simulink model "CryoDetMultiChan_CMB"  (R2016b)
settings: Solver=ode45  StartTime=0.0  StopTime=1000e-6  MaxStep=Tclk/4  RelTol=1e-3
values from neighbouring files (symbols this model uses):
  ds_axi = 16    [setupCryoFPGA_CMB.m]
  Fclk = Fadc    (= 307200000)    [setupCryoFPGA.m]    (also in setupCryoFPGA_CMB.m; setupCryoFPGAorig.m = 312500000)
  notch = tf( [1 a*wNotch/Q wNotch^2], [1 wNotch/Q wNotch^2])    [setupCryoFPGA.m]    (also in setupCryoFPGA_CMB.m; setupCryoFPGAorig.m)
  notch2 = tf( [1 a*wNotch/Q wNotch^2], [1 wNotch/Q wNotch^2])    [setupCryoFPGA.m]    (also in setupCryoFPGA_CMB.m; setupCryoFPGAorig.m)
  notch3 = tf( [1 a*wNotch/Q wNotch^2], [1 wNotch/Q wNotch^2])    [setupCryoFPGA.m]    (also in setupCryoFPGA_CMB.m; setupCryoFPGAorig.m)
  notch4 = tf( [1 a*wNotch/Q wNotch^2], [1 wNotch/Q wNotch^2])    [setupCryoFPGA.m]    (also in setupCryoFPGA_CMB.m; setupCryoFPGAorig.m)
  Tclk = 1/Fclk    (= 3.25520833333e-09)    [setupCryoFPGA.m]    (also in setupCryoFPGA_CMB.m; setupCryoFPGAorig.m = 3.2e-09)
  Ts = 1/Fadc    (= 3.25520833333e-09)    [setupCryoFPGA.m]    (also in setupCryoFPGA_CMB.m; setupCryoFPGAorig.m = 3.2e-09)
undefined symbols (not defined in the file or in its folder): AXI4, i, Lite, xlipgetpartsetting
libraries: xbsIndex_r4 x2077, CryoDetLib x32, hdlsllib x6, simulink x3
(part 11 of 15)

== system CryoDetMultiChan_CMB/DspCore/FTA_Ch0/SixteenLineUDC 0/oneLineUpDown2 ==
  note: `
  note: Delta-F
  note: When synchIn == Addr then reset CIC filters
  note: Turn off this channel if Frequency is 0 or Fnyquist
  note: first data comes out 31 ticks after release of reset
  note: should we tag data with channel number (from addr) and tvalid?
      | This could help synchronize (and debug) next stage decimator
  note: Latch phase advance for interleave at 1/614.4MHz
  note: Decimated_mxREF_QI
  note: Decimated_mxREF_Q
  note: Decimated_mxADC_I
  note: Decimated_mxADC_Q
  note: DAC 1
  note: DAC 0
  note: Downconverter
  note: Downmixed & Decmiated SIG & REF IQ to Output Mux for interleaving
  note: Phase CICs so outputs for different lines interleave; this is done so by timing the CIC reset operation between line channels
  note: 1/614.4MHz phase advance
  note: Digital LO for one resonator
  note: Upconverter
  note: Multiply Signal & Reference
      | by complex LO
      | Note: we don't need dPhi here b/c its not interleaved
  note: mixed_ADC_Q
  note: mixed_ADC_I
  note: mixed_REF_Q
  note: mixed_REF_I
  note: Address
  note: mixed_dec_ADC_IQ
  note: mixed_dec_REF_IQ
  note: LO + Phi Q
  note: LO + Phi I
  note: Complex multiply adds the phase advance to the output frequency per sample:
      |
      | e^jwt x e^jphi = e^j(wt+phi)
  note: Multipliers are for
      | Amplitude Scaling
  note: LO & LO+phi to DAC sum block
  ADC_IQ_in : Inport
  addrIn : Inport  Port=2
  synchIn : Inport  Port=3
  REF_IQ_in1 : Inport  Port=4
  Bus Creator : BusCreator  Inputs=4
  Bus Selector : BusSelector  OutputSignals=channel,dPhiQ,dPhiI
  CIC Compiler 4.0 {,1..3} (4 alike) : xbsIndex_r4/CIC Compiler 4.0   filter_type=Decimation  number_of_stages=3  differential_delay=1  number_of_channels=1  sample_rate_changes=Fixed  fixed_or_initial_rate=16  minimum_rate=16  maximum_rate=16  ratespecification=Sample_Period  sampleperiod=1  hardwareoversamplingrate=1  quantization=Truncation  output_data_width=20  use_xtreme_dsp_slice=off  use_streaming_interface=on  has_aclken=off  has_aresetn=on  has_dout_tready=off  trim_axipin_name=on  gui_behaviour=Sysgen_GUI  input_data_width=18  ip_name=CIC Compiler  ip_version=4.0  dsptool_ready=true  wrapper_available=true  port_translation_map={ 'aclken' => 'en', 'aresetn' => 'rst' }  ipcore_xco_need_fpga_part=true  ipcore_verbose=false  block_type=cic_compiler_v4_0
  Complex Multiplier 6.0 1 : xbsIndex_r4/Complex Multiplier 6.0   hasatlast=off  hasatuser=off  atuserwidth=1  hasbtlast=off  hasbtuser=off  btuserwidth=1  multtype=Use_Mults  optimizegoal=Resources  flowcontrol=NonBlocking  outputwidth=18  roundmode=Truncate  hasctrltlast=off  hasctrltuser=off  ctrltuserwidth=1  outtlastbehv=Null  latencyconfig=Manual  minimumlatency=6  aclken=off  aresetn=off  trim_axipin_name=on  simulation_type=hybrid_sim  simulation_model=sysgen:cmpy_v6_0  data_path_portlist={ 's_axis_a_tdata_real', 's_axis_a_tdata_imag', 's_axis_b_tdata_real', 's_axis_b_tdata_imag', 's_axis_ctrl_tdata_rounding_bit', 'm_axis_dout_tdata_real', 'm_axis_dout_tdata_imag' }  aportwidth=63  bportwidth=63  ip_name=Complex Multiplier  ip_version=6.0  dsptool_ready=true  ipcore_usecache=true  ipcore_useipmodelcache=true  ipcore_verbose=false  ipcore_latency_parameter='minimumlatency'  wrapper_available=true  port_translation_map={ 'aclken' => 'en', 'aresetn' => 'rst'}  block_type=cmpy_v6_0
  Complex Multiplier 6.0 2 : xbsIndex_r4/Complex Multiplier 6.0   hasatlast=off  hasatuser=off  atuserwidth=1  hasbtlast=off  hasbtuser=off  btuserwidth=1  multtype=Use_Mults  optimizegoal=Resources  flowcontrol=NonBlocking  outputwidth=18  roundmode=Truncate  hasctrltlast=off  hasctrltuser=off  ctrltuserwidth=1  outtlastbehv=Null  latencyconfig=Manual  minimumlatency=6  aclken=off  aresetn=off  trim_axipin_name=on  simulation_type=hybrid_sim  simulation_model=sysgen:cmpy_v6_0  data_path_portlist={ 's_axis_a_tdata_real', 's_axis_a_tdata_imag', 's_axis_b_tdata_real', 's_axis_b_tdata_imag', 's_axis_ctrl_tdata_rounding_bit', 'm_axis_dout_tdata_real', 'm_axis_dout_tdata_imag' }  aportwidth=63  bportwidth=63  ip_name=Complex Multiplier  ip_version=6.0  dsptool_ready=true  ipcore_usecache=true  ipcore_useipmodelcache=true  ipcore_verbose=false  ipcore_latency_parameter='minimumlatency'  wrapper_available=true  port_translation_map={ 'aclken' => 'en', 'aresetn' => 'rst'}  block_type=cmpy_v6_0
  Complex Multiplier 6.0 4 : xbsIndex_r4/Complex Multiplier 6.0   hasatlast=off  hasatuser=off  atuserwidth=1  hasbtlast=off  hasbtuser=off  btuserwidth=1  multtype=Use_Mults  optimizegoal=Resources  flowcontrol=NonBlocking  outputwidth=19  roundmode=Truncate  hasctrltlast=off  hasctrltuser=off  ctrltuserwidth=1  outtlastbehv=Null  latencyconfig=Manual  minimumlatency=6  aclken=off  aresetn=off  trim_axipin_name=on  simulation_type=hybrid_sim  simulation_model=sysgen:cmpy_v6_0  data_path_portlist={ 's_axis_a_tdata_real', 's_axis_a_tdata_imag', 's_axis_b_tdata_real', 's_axis_b_tdata_imag', 's_axis_ctrl_tdata_rounding_bit', 'm_axis_dout_tdata_real', 'm_axis_dout_tdata_imag' }  aportwidth=63  bportwidth=63  ip_name=Complex Multiplier  ip_version=6.0  dsptool_ready=true  ipcore_usecache=true  ipcore_useipmodelcache=true  ipcore_verbose=false  ipcore_latency_parameter='minimumlatency'  wrapper_available=true  port_translation_map={ 'aclken' => 'en', 'aresetn' => 'rst'}  block_type=cmpy_v6_0
  Constant : xbsIndex_r4/Constant  const=1  gui_display_data_type=Boolean  arith_type=Boolean  n_bits=16  bin_pt=14  preci_type=Single  exp_width=8  frac_width=24  explicit_period=on  period=Tclk  equ=P=C  opselect=C  inp2=PCIN>>17  opr=+  inp1=P  carry=CIN  dbl_ovrd=off  block_type=constant
  Constant1 : xbsIndex_r4/Constant  const=0  gui_display_data_type=Fixed-point  arith_type=Unsigned  n_bits=16  bin_pt=16  preci_type=Single  exp_width=8  frac_width=24  explicit_period=off  period=1  equ=P=C  opselect=C  inp2=PCIN>>17  opr=+  inp1=P  carry=CIN  dbl_ovrd=off  block_type=constant
  Constant2 : xbsIndex_r4/Constant  const=0  gui_display_data_type=Fixed-point  arith_type=Unsigned  n_bits=16  bin_pt=16  preci_type=Single  exp_width=8  frac_width=24  explicit_period=off  period=1  equ=P=C  opselect=C  inp2=PCIN>>17  opr=+  inp1=P  carry=CIN  dbl_ovrd=off  block_type=constant
  Constant3 : xbsIndex_r4/Constant  const=1  gui_display_data_type=Boolean  arith_type=Boolean  n_bits=16  bin_pt=14  preci_type=Single  exp_width=8  frac_width=24  explicit_period=on  period=Tclk  equ=P=C  opselect=C  inp2=PCIN>>17  opr=+  inp1=P  carry=CIN  dbl_ovrd=off  block_type=constant
  Convert1 : xbsIndex_r4/Convert  gui_display_data_type=Fixed-point  arith_type="Signed  (2's comp)"  n_bits=16  bin_pt=14  float_type=Single  exp_bits=8  fraction_bits=24  quantization=Truncate  overflow=Saturate  en=off  latency=1  pipeline=off  dbl_ovrd=off  block_type=convert
  Convert2 : xbsIndex_r4/Convert  gui_display_data_type=Fixed-point  arith_type="Signed  (2's comp)"  n_bits=16  bin_pt=14  float_type=Single  exp_bits=8  fraction_bits=24  quantization=Truncate  overflow=Saturate  en=off  latency=1  pipeline=off  dbl_ovrd=off  block_type=convert
  Counter : xbsIndex_r4/Counter  cnt_type=Free Running  cnt_to=Inf  operation=Up  start_count=0  cnt_by_val=1  arith_type=Unsigned  n_bits=8  bin_pt=0  load_pin=off  rst=on  en=off  explicit_period=off  period=1  use_behavioral_HDL=off  implementation=Fabric  dbl_ovrd=off  block_type=counter
  "DDS Compiler 6.0 " : xbsIndex_r4/DDS Compiler 6.0   partspresent=Phase_Generator_and_SIN_COS_LUT  dds_clock_rate=Fclk/1e6  channels=1  mode_of_operation=Standard  modulus=9  parameter_entry=Hardware_Parameters  spurious_free_dynamic_range=36.00000000  frequency_resolution=0.40000000  noise_shaping=None  phase_width=freqBits  output_width=IQbits  output_selection=Sine_and_Cosine  negative_sine=off  negative_cosine=off  amplitude_mode=Unit_Circle  memory_type=Auto  optimization_goal=Speed  dsp48_use=Maximal  resync=off  latency_configuration=Configurable  latency=15  has_phase_out=off  has_aclken=off  has_aresetn=off  explicit_period=on  period=Tclk  data_has_tlast=Not_Required  has_tready=off  s_phase_has_tuser=Not_Required  m_data_has_tuser=Not_Required  m_phase_has_tuser=Not_Required  s_phase_tuser_width=1  output_form=Twos_Complement  s_config_sync_mode=On_Vector  phase_increment=Programmable  output_frequency1=0  output_frequency2=0  output_frequency3=0  output_frequency4=0  output_frequency5=0  output_frequency6=0  output_frequency7=0  output_frequency8=0  output_frequency9=0  output_frequency10=0  output_frequency11=0  output_frequency12=0  output_frequency13=0  output_frequency14=0  output_frequency15=0  output_frequency16=0  pinc1='0'  pinc2='0'  pinc3='0'  pinc4='0'  pinc5='0'  pinc6='0'  pinc7='0'  pinc8='0'  pinc9='0'  pinc10='0'  pinc11='0'  pinc12='0'  pinc13='0'  pinc14='0'  pinc15='0'  pinc16='0'  phase_offset=None  phase_offset_angles1=0  phase_offset_angles2=0  phase_offset_angles3=0  phase_offset_angles4=0  phase_offset_angles5=0  phase_offset_angles6=0  phase_offset_angles7=0  phase_offset_angles8=0  phase_offset_angles9=0  phase_offset_angles10=0  phase_offset_angles11=0  phase_offset_angles12=0  phase_offset_angles13=0  phase_offset_angles14=0  phase_offset_angles15=0  phase_offset_angles16=0  poff1='0'  poff2='0'  poff3='0'  poff4='0'  poff5='0'  poff6='0'  poff7='0'  poff8='0'  poff9='0'  poff10='0'  poff11='0'  poff12='0'  poff13='0'  poff14='0'  poff15='0'  poff16='0'  trim_axipin_name=on  simulation_type=hybrid_sim  simulation_model=sysgen:xddsv6_0_cmodel  data_path_portlist={ 's_axis_config_tdata_poff', 's_axis_config_tdata_chan0_poff', 's_axis_config_tdata_pinc', 's_axis_config_tdata_chan0_pinc', 's_axis_phase_tdata_resync', 's_axis_phase_tdata_chan0_resync', 's_axis_phase_tdata_poff', 's_axis_phase_tdata_chan0_poff', 's_axis_phase_tdata_pinc', 's_axis_phase_tdata_chan0_pinc', 's_axis_phase_tdata_phase_in', 'm_axis_data_tdata_sine', 'm_axis_data_tdata_chan0_sine', 'm_axis_data_tdata_cosine', 'm_axis_data_tdata_chan0_cosine', 'm_axis_phase_tdata_phase_out', 'm_axis_phase_tdata_chan0_phase_out'}  por_mode=false  gui_behaviour=Sysgen  ip_name=DDS Compiler  ip_version=6.0  dsptool_ready=true  wrapper_available=true  port_translation_map={ 'aclken' => 'en', 'aresetn' => 'rst' }  ipcore_usecache=true  ipcore_useipmodelcache=true  ipcore_xco_need_fpga_part=true  ipcore_fpga_part=xlipgetpartsetting(gcb, {'kintex7', 'xc7k325t', '-3', 'fbg676'})  ipcore_verbose=false  block_type=dds_compiler_v6_0
  DLO1 scope : Scope  NumInputPorts=2
  DLO1 scope1 : Scope  NumInputPorts=2
  Delay : xbsIndex_r4/Delay  rst=off  infoeditControl=Selection of Reset will increase slice count due to use of real FFs and instead of SRLs  en=off  latency=7  reg_retiming=off  dbl_ovrd=off  block_type=delay
  Delay1 : xbsIndex_r4/Delay  rst=off  infoeditControl=Selection of Reset will increase slice count due to use of real FFs and instead of SRLs  en=off  latency=7  reg_retiming=on  dbl_ovrd=off  block_type=delay
  Demux1 : Demux
  Demux2 : Demux  Outputs=2
  Demux3 : Demux  Outputs=2
  Display3 : Display
  Display4 : Display
  Display5 : Display
  Gateway Out{1..31} (31 alike) : xbsIndex_r4/Gateway Out  inherit_from_input=off  hdl_port=off  rows=1  columns=1  UseAsDAC=off  DACChannel='1'  interface=None  automatic_assignment=on  address_offset=hex2dec('00')  intf_name=''  intf_description=''  timing_constraint=None  locs_specified=off  LOCs={}  io_standard={}  block_type=gatewayout
  Inverter : xbsIndex_r4/Inverter  en=off  latency=0  dbl_ovrd=off  block_type=inv
  Mult{1..2,8..9} (4 alike) : xbsIndex_r4/Mult  precision=User Defined  arith_type="Signed  (2's comp)"  n_bits=16  bin_pt=15  quantization=Truncate  overflow=Wrap  en=off  latency=3  use_behavioral_HDL=off  opt=Speed  use_embedded=on  optimum_pipeline=off  pipeline=on  dbl_ovrd=off  use_rpm=on  placement_style=Triangular  block_type=mult
  Mux{,1..8} (9 alike) : Mux  Inputs=2
  Mux13 : xbsIndex_r4/Mux  inputs=2  en=off  latency=0  precision=Full  arith_type=Unsigned  n_bits=16  bin_pt=14  quantization=Truncate  overflow=Wrap  dbl_ovrd=off  block_type=mux
  Register : xbsIndex_r4/Register  init=0  rst=off  en=on  dbl_ovrd=off  block_type=register
  Register1 : xbsIndex_r4/Register  init=0  rst=off  en=on  dbl_ovrd=off  block_type=register
  Register{3..9} (7 alike) : xbsIndex_r4/Register  init=0  rst=off  en=off  dbl_ovrd=off  block_type=register
  Reinterpret2 : xbsIndex_r4/Reinterpret  force_arith_type=on  arith_type=Unsigned  force_bin_pt=on  bin_pt=freqBits  block_type=reinterpret
  Relational : xbsIndex_r4/Relational  mode=a=b  op_type=Bool  en=off  latency=0  dbl_ovrd=off  block_type=relational
  Relational1 : xbsIndex_r4/Relational  mode=a=b  op_type=Bool  en=off  latency=0  dbl_ovrd=off  block_type=relational
  Relational2 : xbsIndex_r4/Relational  mode=a!=b  op_type=Ufix  en=off  latency=1  dbl_ovrd=off  block_type=relational
  Relational3 : xbsIndex_r4/Relational  mode=a!=b  op_type=Bool  en=off  latency=0  dbl_ovrd=off  block_type=relational
  Scale{1..4} (4 alike) : xbsIndex_r4/Scale  scale_factor=-12  dbl_ovrd=off  block_type=scale
  Slice : xbsIndex_r4/Slice  nbits=freqBusAddrBits  boolean_output=off  mode=Lower Bit Location + Width  bit1=0  base1=MSB of Input  bit0=freqBits  base0=LSB of Input  dbl_ovrd=off  block_type=slice
  Slice1 : xbsIndex_r4/Slice  nbits=freqBits  boolean_output=off  mode=Lower Bit Location + Width  bit1=0  base1=MSB of Input  bit0=0  base0=LSB of Input  dbl_ovrd=off  block_type=slice
  Terminator{,1..6,8} (8 alike) : Terminator
  block downconverter Scope : Scope  NumInputPorts=3
  block downconverter Scope1 : Scope  NumInputPorts=2
  block downconverter Scope2 : Scope  NumInputPorts=6
  block downconverter Scope3 : Scope  NumInputPorts=8
  DC_Out : Outport
  UC_out : Outport  Port=2
  wires:
  Relational/1 -> "DDS Compiler 6.0 "/1
  [freqBus] -> Register3/1
  Slice/1 -> Relational/2
  Slice1/1 -> Reinterpret2/1
  addrIn/1 -> [Addr], Relational1/1, Relational/1
  "DDS Compiler 6.0 "/2 -> Complex Multiplier 6.0 4/2, Delay/1
  "DDS Compiler 6.0 "/3 -> Complex Multiplier 6.0 4/3, Delay1/1
  Relational1/1 -> Register/2, Register1/2
  Register1/1 -> Gateway Out15/1, Complex Multiplier 6.0 4/6
  Register/1 -> Relational2/2, Gateway Out16/1, Complex Multiplier 6.0 4/5
  "DDS Compiler 6.0 "/1 -> Complex Multiplier 6.0 4/1, Complex Multiplier 6.0 4/4
  Delay/1 -> Mult1/1, Gateway Out8/1, [UC_LO_Q]
  Delay1/1 -> Gateway Out7/1, Mult8/1, [UC_LO_I]
  "CIC Compiler 4.0 "/3 -> Gateway Out31/1, Scale1/1
  CIC Compiler 4.0 3/3 -> Scale4/1
  CIC Compiler 4.0 2/3 -> Scale3/1
  CIC Compiler 4.0 1/3 -> Gateway Out30/1, Scale2/1
  Mux2/1 -> Demux1/1, DC_Out/1
  Scale4/1 -> Gateway Out13/1, Mux1/2  "mdREF_I"
  Scale3/1 -> Gateway Out14/1, Mux1/1  "mdREF_Q"
  Scale2/1 -> Mux/2  "mdADC_I"
  Scale1/1 -> Mux/1  "mdADC_Q"
  Constant/1 -> CIC Compiler 4.0 1/1, CIC Compiler 4.0 3/1, CIC Compiler 4.0 2/1, "CIC Compiler 4.0 "/1
  Mux1/1 -> Mux2/2
  Mux/1 -> Mux2/1
  "CIC Compiler 4.0 "/1 -> Terminator/1
  CIC Compiler 4.0 1/1 -> Terminator2/1
  CIC Compiler 4.0 1/2 -> Terminator3/1
  CIC Compiler 4.0 2/1 -> Terminator4/1
  CIC Compiler 4.0 2/2 -> Terminator5/1
  Complex Multiplier 6.0 4/1 -> Terminator8/1
  Bus Selector/2 -> Register/1  "<dPhiQ>"
  Bus Selector/3 -> Register1/1  "<dPhiI>"
  Reinterpret2/1 -> "DDS Compiler 6.0 "/2
  [dphiBus] -> Bus Selector/1
  Bus Selector/1 -> Relational1/2  "<channel>"
  Demux1/1 -> Gateway Out3/1
  Demux1/2 -> Gateway Out4/1
  Demux1/3 -> Gateway Out5/1
  Demux1/4 -> Gateway Out6/1
  Gateway Out6/1 -> Mux5/2
  Gateway Out5/1 -> Mux5/1
  Gateway Out4/1 -> Mux4/2
  Gateway Out3/1 -> Mux4/1
  Mux4/1 -> block downconverter Scope/1
  Mux5/1 -> block downconverter Scope/2
  Convert2/1 -> Gateway Out9/1, Mult9/2
  Convert1/1 -> Gateway Out10/1, Mult2/2
  Gateway Out10/1 -> Mux7/2
  Gateway Out9/1 -> Mux7/1
  Gateway Out8/1 -> Mux6/2
  Gateway Out7/1 -> Mux6/1
  Mux6/1 -> DLO1 scope/1
  Mux7/1 -> DLO1 scope/2
  Gateway Out16/1 -> Display4/1
  Gateway Out15/1 -> Display3/1
  Constant1/1 -> Mux13/2
  [Ampl0] -> Mux13/3
  Mux13/1 -> Gateway Out20/1, Mult9/1, Mult2/1, Mult1/2, Mult8/2
  Constant2/1 -> Relational2/1
  Relational2/1 -> Mux13/1
  Gateway Out20/1 -> Display5/1
  Relational3/1 -> Inverter/1, "CIC Compiler 4.0 "/3, CIC Compiler 4.0 1/3, CIC Compiler 4.0 3/3, CIC Compiler 4.0 2/3
  [Addr] -> Relational3/2
  synchIn/1 -> Relational3/1
  Gateway Out21/1 -> block downconverter Scope1/1
  Counter/1 -> Gateway Out22/1
  Gateway Out22/1 -> block downconverter Scope/3, block downconverter Scope1/2
  Inverter/1 -> Counter/1, Gateway Out21/1
  ADC_IQ_in/1 -> Demux2/1
  Demux2/1 -> Gateway Out29/1, Complex Multiplier 6.0 1/2
  Demux2/2 -> Gateway Out24/1, Complex Multiplier 6.0 1/3
  Complex Multiplier 6.0 1/2 -> "CIC Compiler 4.0 "/2, Gateway Out28/1
  Complex Multiplier 6.0 1/3 -> Gateway Out27/1, CIC Compiler 4.0 1/2
  [UC_LO_Q] -> Gateway Out26/1, Complex Multiplier 6.0 2/5, Complex Multiplier 6.0 1/5
  [UC_LO_I] -> Gateway Out25/1, Complex Multiplier 6.0 2/6, Complex Multiplier 6.0 1/6
  Complex Multiplier 6.0 2/3 -> CIC Compiler 4.0 3/2, Gateway Out12/1
  Complex Multiplier 6.0 2/2 -> CIC Compiler 4.0 2/2, Gateway Out11/1
  Demux3/1 -> Register8/1
  Demux3/2 -> Register9/1
  REF_IQ_in1/1 -> Demux3/1
  Constant3/1 -> Complex Multiplier 6.0 1/1, Complex Multiplier 6.0 1/4, Complex Multiplier 6.0 2/4, Complex Multiplier 6.0 2/1
  CIC Compiler 4.0 3/1 -> Terminator1/1
  CIC Compiler 4.0 3/2 -> Terminator6/1
  Mult1/1 -> Register7/1, Gateway Out19/1
  Mult8/1 -> Register6/1, Gateway Out18/1
  Mult2/1 -> Register5/1, Gateway Out17/1
  Mult9/1 -> Register4/1, Gateway Out23/1
  Mux3/1 -> DLO1 scope1/1
  Mux8/1 -> DLO1 scope1/2
  Complex Multiplier 6.0 4/3 -> Convert2/1
  Complex Multiplier 6.0 4/2 -> Convert1/1
  Gateway Out1/1 -> block downconverter Scope2/1
  Gateway Out2/1 -> block downconverter Scope2/2
  Gateway Out11/1 -> block downconverter Scope2/3
  Gateway Out12/1 -> block downconverter Scope2/4
  Gateway Out13/1 -> block downconverter Scope2/5
  Gateway Out14/1 -> block downconverter Scope2/6
  Gateway Out17/1 -> Mux8/2
  Gateway Out23/1 -> Mux8/1
  Gateway Out19/1 -> Mux3/2
  Gateway Out18/1 -> Mux3/1
  Gateway Out24/1 -> block downconverter Scope3/1
  Gateway Out29/1 -> block downconverter Scope3/2
  Gateway Out25/1 -> block downconverter Scope3/3
  Gateway Out26/1 -> block downconverter Scope3/4
  Gateway Out27/1 -> block downconverter Scope3/5
  Gateway Out28/1 -> block downconverter Scope3/6
  Gateway Out30/1 -> block downconverter Scope3/7
  Gateway Out31/1 -> block downconverter Scope3/8
  Register3/1 -> Slice1/1, Slice/1
  Register8/1 -> Gateway Out2/1, Complex Multiplier 6.0 2/2
  Register9/1 -> Gateway Out1/1, Complex Multiplier 6.0 2/3
  Bus Creator/1 -> UC_out/1
  Register4/1 -> Bus Creator/4  "UC_out_Ip"
  Register5/1 -> Bus Creator/3  "UC_out_Qp"
  Register6/1 -> Bus Creator/2  "UC_out_I"
  Register7/1 -> Bus Creator/1  "UC_out_Q"

== system CryoDetMultiChan_CMB/DspCore/FTA_Ch0/SixteenLineUDC 0/oneLineUpDown3 ==
  note: `
  note: Delta-F
  note: When synchIn == Addr then reset CIC filters
  note: Turn off this channel if Frequency is 0 or Fnyquist
  note: first data comes out 31 ticks after release of reset
  note: should we tag data with channel number (from addr) and tvalid?
      | This could help synchronize (and debug) next stage decimator
  note: Latch phase advance for interleave at 1/614.4MHz
  note: Decimated_mxREF_QI
  note: Decimated_mxREF_Q
  note: Decimated_mxADC_I
  note: Decimated_mxADC_Q
  note: DAC 1
  note: DAC 0
  note: Downconverter
  note: Downmixed & Decmiated SIG & REF IQ to Output Mux for interleaving
  note: Phase CICs so outputs for different lines interleave; this is done so by timing the CIC reset operation between line channels
  note: 1/614.4MHz phase advance
  note: Digital LO for one resonator
  note: Upconverter
  note: Multiply Signal & Reference
      | by complex LO
      | Note: we don't need dPhi here b/c its not interleaved
  note: mixed_ADC_Q
  note: mixed_ADC_I
  note: mixed_REF_Q
  note: mixed_REF_I
  note: Address
  note: mixed_dec_ADC_IQ
  note: mixed_dec_REF_IQ
  note: LO + Phi Q
  note: LO + Phi I
  note: Complex multiply adds the phase advance to the output frequency per sample:
      |
      | e^jwt x e^jphi = e^j(wt+phi)
  note: Multipliers are for
      | Amplitude Scaling
  note: LO & LO+phi to DAC sum block
  ADC_IQ_in : Inport
  addrIn : Inport  Port=2
  synchIn : Inport  Port=3
  REF_IQ_in1 : Inport  Port=4
  Bus Creator : BusCreator  Inputs=4
  Bus Selector : BusSelector  OutputSignals=channel,dPhiQ,dPhiI
  CIC Compiler 4.0 {,1..3} (4 alike) : xbsIndex_r4/CIC Compiler 4.0   filter_type=Decimation  number_of_stages=3  differential_delay=1  number_of_channels=1  sample_rate_changes=Fixed  fixed_or_initial_rate=16  minimum_rate=16  maximum_rate=16  ratespecification=Sample_Period  sampleperiod=1  hardwareoversamplingrate=1  quantization=Truncation  output_data_width=20  use_xtreme_dsp_slice=off  use_streaming_interface=on  has_aclken=off  has_aresetn=on  has_dout_tready=off  trim_axipin_name=on  gui_behaviour=Sysgen_GUI  input_data_width=18  ip_name=CIC Compiler  ip_version=4.0  dsptool_ready=true  wrapper_available=true  port_translation_map={ 'aclken' => 'en', 'aresetn' => 'rst' }  ipcore_xco_need_fpga_part=true  ipcore_verbose=false  block_type=cic_compiler_v4_0
  Complex Multiplier 6.0 1 : xbsIndex_r4/Complex Multiplier 6.0   hasatlast=off  hasatuser=off  atuserwidth=1  hasbtlast=off  hasbtuser=off  btuserwidth=1  multtype=Use_Mults  optimizegoal=Resources  flowcontrol=NonBlocking  outputwidth=18  roundmode=Truncate  hasctrltlast=off  hasctrltuser=off  ctrltuserwidth=1  outtlastbehv=Null  latencyconfig=Manual  minimumlatency=6  aclken=off  aresetn=off  trim_axipin_name=on  simulation_type=hybrid_sim  simulation_model=sysgen:cmpy_v6_0  data_path_portlist={ 's_axis_a_tdata_real', 's_axis_a_tdata_imag', 's_axis_b_tdata_real', 's_axis_b_tdata_imag', 's_axis_ctrl_tdata_rounding_bit', 'm_axis_dout_tdata_real', 'm_axis_dout_tdata_imag' }  aportwidth=63  bportwidth=63  ip_name=Complex Multiplier  ip_version=6.0  dsptool_ready=true  ipcore_usecache=true  ipcore_useipmodelcache=true  ipcore_verbose=false  ipcore_latency_parameter='minimumlatency'  wrapper_available=true  port_translation_map={ 'aclken' => 'en', 'aresetn' => 'rst'}  block_type=cmpy_v6_0
  Complex Multiplier 6.0 2 : xbsIndex_r4/Complex Multiplier 6.0   hasatlast=off  hasatuser=off  atuserwidth=1  hasbtlast=off  hasbtuser=off  btuserwidth=1  multtype=Use_Mults  optimizegoal=Resources  flowcontrol=NonBlocking  outputwidth=18  roundmode=Truncate  hasctrltlast=off  hasctrltuser=off  ctrltuserwidth=1  outtlastbehv=Null  latencyconfig=Manual  minimumlatency=6  aclken=off  aresetn=off  trim_axipin_name=on  simulation_type=hybrid_sim  simulation_model=sysgen:cmpy_v6_0  data_path_portlist={ 's_axis_a_tdata_real', 's_axis_a_tdata_imag', 's_axis_b_tdata_real', 's_axis_b_tdata_imag', 's_axis_ctrl_tdata_rounding_bit', 'm_axis_dout_tdata_real', 'm_axis_dout_tdata_imag' }  aportwidth=63  bportwidth=63  ip_name=Complex Multiplier  ip_version=6.0  dsptool_ready=true  ipcore_usecache=true  ipcore_useipmodelcache=true  ipcore_verbose=false  ipcore_latency_parameter='minimumlatency'  wrapper_available=true  port_translation_map={ 'aclken' => 'en', 'aresetn' => 'rst'}  block_type=cmpy_v6_0
  Complex Multiplier 6.0 4 : xbsIndex_r4/Complex Multiplier 6.0   hasatlast=off  hasatuser=off  atuserwidth=1  hasbtlast=off  hasbtuser=off  btuserwidth=1  multtype=Use_Mults  optimizegoal=Resources  flowcontrol=NonBlocking  outputwidth=19  roundmode=Truncate  hasctrltlast=off  hasctrltuser=off  ctrltuserwidth=1  outtlastbehv=Null  latencyconfig=Manual  minimumlatency=6  aclken=off  aresetn=off  trim_axipin_name=on  simulation_type=hybrid_sim  simulation_model=sysgen:cmpy_v6_0  data_path_portlist={ 's_axis_a_tdata_real', 's_axis_a_tdata_imag', 's_axis_b_tdata_real', 's_axis_b_tdata_imag', 's_axis_ctrl_tdata_rounding_bit', 'm_axis_dout_tdata_real', 'm_axis_dout_tdata_imag' }  aportwidth=63  bportwidth=63  ip_name=Complex Multiplier  ip_version=6.0  dsptool_ready=true  ipcore_usecache=true  ipcore_useipmodelcache=true  ipcore_verbose=false  ipcore_latency_parameter='minimumlatency'  wrapper_available=true  port_translation_map={ 'aclken' => 'en', 'aresetn' => 'rst'}  block_type=cmpy_v6_0
  Constant : xbsIndex_r4/Constant  const=1  gui_display_data_type=Boolean  arith_type=Boolean  n_bits=16  bin_pt=14  preci_type=Single  exp_width=8  frac_width=24  explicit_period=on  period=Tclk  equ=P=C  opselect=C  inp2=PCIN>>17  opr=+  inp1=P  carry=CIN  dbl_ovrd=off  block_type=constant
  Constant1 : xbsIndex_r4/Constant  const=0  gui_display_data_type=Fixed-point  arith_type=Unsigned  n_bits=16  bin_pt=16  preci_type=Single  exp_width=8  frac_width=24  explicit_period=off  period=1  equ=P=C  opselect=C  inp2=PCIN>>17  opr=+  inp1=P  carry=CIN  dbl_ovrd=off  block_type=constant
  Constant2 : xbsIndex_r4/Constant  const=0  gui_display_data_type=Fixed-point  arith_type=Unsigned  n_bits=16  bin_pt=16  preci_type=Single  exp_width=8  frac_width=24  explicit_period=off  period=1  equ=P=C  opselect=C  inp2=PCIN>>17  opr=+  inp1=P  carry=CIN  dbl_ovrd=off  block_type=constant
  Constant3 : xbsIndex_r4/Constant  const=1  gui_display_data_type=Boolean  arith_type=Boolean  n_bits=16  bin_pt=14  preci_type=Single  exp_width=8  frac_width=24  explicit_period=on  period=Tclk  equ=P=C  opselect=C  inp2=PCIN>>17  opr=+  inp1=P  carry=CIN  dbl_ovrd=off  block_type=constant
  Convert1 : xbsIndex_r4/Convert  gui_display_data_type=Fixed-point  arith_type="Signed  (2's comp)"  n_bits=16  bin_pt=14  float_type=Single  exp_bits=8  fraction_bits=24  quantization=Truncate  overflow=Saturate  en=off  latency=1  pipeline=off  dbl_ovrd=off  block_type=convert
  Convert2 : xbsIndex_r4/Convert  gui_display_data_type=Fixed-point  arith_type="Signed  (2's comp)"  n_bits=16  bin_pt=14  float_type=Single  exp_bits=8  fraction_bits=24  quantization=Truncate  overflow=Saturate  en=off  latency=1  pipeline=off  dbl_ovrd=off  block_type=convert
  Counter : xbsIndex_r4/Counter  cnt_type=Free Running  cnt_to=Inf  operation=Up  start_count=0  cnt_by_val=1  arith_type=Unsigned  n_bits=8  bin_pt=0  load_pin=off  rst=on  en=off  explicit_period=off  period=1  use_behavioral_HDL=off  implementation=Fabric  dbl_ovrd=off  block_type=counter
  "DDS Compiler 6.0 " : xbsIndex_r4/DDS Compiler 6.0   partspresent=Phase_Generator_and_SIN_COS_LUT  dds_clock_rate=Fclk/1e6  channels=1  mode_of_operation=Standard  modulus=9  parameter_entry=Hardware_Parameters  spurious_free_dynamic_range=36.00000000  frequency_resolution=0.40000000  noise_shaping=None  phase_width=freqBits  output_width=IQbits  output_selection=Sine_and_Cosine  negative_sine=off  negative_cosine=off  amplitude_mode=Unit_Circle  memory_type=Auto  optimization_goal=Speed  dsp48_use=Maximal  resync=off  latency_configuration=Configurable  latency=15  has_phase_out=off  has_aclken=off  has_aresetn=off  explicit_period=on  period=Tclk  data_has_tlast=Not_Required  has_tready=off  s_phase_has_tuser=Not_Required  m_data_has_tuser=Not_Required  m_phase_has_tuser=Not_Required  s_phase_tuser_width=1  output_form=Twos_Complement  s_config_sync_mode=On_Vector  phase_increment=Programmable  output_frequency1=0  output_frequency2=0  output_frequency3=0  output_frequency4=0  output_frequency5=0  output_frequency6=0  output_frequency7=0  output_frequency8=0  output_frequency9=0  output_frequency10=0  output_frequency11=0  output_frequency12=0  output_frequency13=0  output_frequency14=0  output_frequency15=0  output_frequency16=0  pinc1='0'  pinc2='0'  pinc3='0'  pinc4='0'  pinc5='0'  pinc6='0'  pinc7='0'  pinc8='0'  pinc9='0'  pinc10='0'  pinc11='0'  pinc12='0'  pinc13='0'  pinc14='0'  pinc15='0'  pinc16='0'  phase_offset=None  phase_offset_angles1=0  phase_offset_angles2=0  phase_offset_angles3=0  phase_offset_angles4=0  phase_offset_angles5=0  phase_offset_angles6=0  phase_offset_angles7=0  phase_offset_angles8=0  phase_offset_angles9=0  phase_offset_angles10=0  phase_offset_angles11=0  phase_offset_angles12=0  phase_offset_angles13=0  phase_offset_angles14=0  phase_offset_angles15=0  phase_offset_angles16=0  poff1='0'  poff2='0'  poff3='0'  poff4='0'  poff5='0'  poff6='0'  poff7='0'  poff8='0'  poff9='0'  poff10='0'  poff11='0'  poff12='0'  poff13='0'  poff14='0'  poff15='0'  poff16='0'  trim_axipin_name=on  simulation_type=hybrid_sim  simulation_model=sysgen:xddsv6_0_cmodel  data_path_portlist={ 's_axis_config_tdata_poff', 's_axis_config_tdata_chan0_poff', 's_axis_config_tdata_pinc', 's_axis_config_tdata_chan0_pinc', 's_axis_phase_tdata_resync', 's_axis_phase_tdata_chan0_resync', 's_axis_phase_tdata_poff', 's_axis_phase_tdata_chan0_poff', 's_axis_phase_tdata_pinc', 's_axis_phase_tdata_chan0_pinc', 's_axis_phase_tdata_phase_in', 'm_axis_data_tdata_sine', 'm_axis_data_tdata_chan0_sine', 'm_axis_data_tdata_cosine', 'm_axis_data_tdata_chan0_cosine', 'm_axis_phase_tdata_phase_out', 'm_axis_phase_tdata_chan0_phase_out'}  por_mode=false  gui_behaviour=Sysgen  ip_name=DDS Compiler  ip_version=6.0  dsptool_ready=true  wrapper_available=true  port_translation_map={ 'aclken' => 'en', 'aresetn' => 'rst' }  ipcore_usecache=true  ipcore_useipmodelcache=true  ipcore_xco_need_fpga_part=true  ipcore_fpga_part=xlipgetpartsetting(gcb, {'kintex7', 'xc7k325t', '-3', 'fbg676'})  ipcore_verbose=false  block_type=dds_compiler_v6_0
  DLO1 scope : Scope  NumInputPorts=2
  DLO1 scope1 : Scope  NumInputPorts=2
  Delay : xbsIndex_r4/Delay  rst=off  infoeditControl=Selection of Reset will increase slice count due to use of real FFs and instead of SRLs  en=off  latency=7  reg_retiming=off  dbl_ovrd=off  block_type=delay
  Delay1 : xbsIndex_r4/Delay  rst=off  infoeditControl=Selection of Reset will increase slice count due to use of real FFs and instead of SRLs  en=off  latency=7  reg_retiming=on  dbl_ovrd=off  block_type=delay
  Demux1 : Demux
  Demux2 : Demux  Outputs=2
  Demux3 : Demux  Outputs=2
  Display3 : Display
  Display4 : Display
  Display5 : Display
  Gateway Out{1..31} (31 alike) : xbsIndex_r4/Gateway Out  inherit_from_input=off  hdl_port=off  rows=1  columns=1  UseAsDAC=off  DACChannel='1'  interface=None  automatic_assignment=on  address_offset=hex2dec('00')  intf_name=''  intf_description=''  timing_constraint=None  locs_specified=off  LOCs={}  io_standard={}  block_type=gatewayout
  Inverter : xbsIndex_r4/Inverter  en=off  latency=0  dbl_ovrd=off  block_type=inv
  Mult{1..2,8..9} (4 alike) : xbsIndex_r4/Mult  precision=User Defined  arith_type="Signed  (2's comp)"  n_bits=16  bin_pt=15  quantization=Truncate  overflow=Wrap  en=off  latency=3  use_behavioral_HDL=off  opt=Speed  use_embedded=on  optimum_pipeline=off  pipeline=on  dbl_ovrd=off  use_rpm=on  placement_style=Triangular  block_type=mult
  Mux{,1..8} (9 alike) : Mux  Inputs=2
  Mux13 : xbsIndex_r4/Mux  inputs=2  en=off  latency=0  precision=Full  arith_type=Unsigned  n_bits=16  bin_pt=14  quantization=Truncate  overflow=Wrap  dbl_ovrd=off  block_type=mux
  Register : xbsIndex_r4/Register  init=0  rst=off  en=on  dbl_ovrd=off  block_type=register
  Register1 : xbsIndex_r4/Register  init=0  rst=off  en=on  dbl_ovrd=off  block_type=register
  Register{3..9} (7 alike) : xbsIndex_r4/Register  init=0  rst=off  en=off  dbl_ovrd=off  block_type=register
  Reinterpret2 : xbsIndex_r4/Reinterpret  force_arith_type=on  arith_type=Unsigned  force_bin_pt=on  bin_pt=freqBits  block_type=reinterpret
  Relational : xbsIndex_r4/Relational  mode=a=b  op_type=Bool  en=off  latency=0  dbl_ovrd=off  block_type=relational
  Relational1 : xbsIndex_r4/Relational  mode=a=b  op_type=Bool  en=off  latency=0  dbl_ovrd=off  block_type=relational
  Relational2 : xbsIndex_r4/Relational  mode=a!=b  op_type=Ufix  en=off  latency=1  dbl_ovrd=off  block_type=relational
  Relational3 : xbsIndex_r4/Relational  mode=a!=b  op_type=Bool  en=off  latency=0  dbl_ovrd=off  block_type=relational
  Scale{1..4} (4 alike) : xbsIndex_r4/Scale  scale_factor=-12  dbl_ovrd=off  block_type=scale
  Slice : xbsIndex_r4/Slice  nbits=freqBusAddrBits  boolean_output=off  mode=Lower Bit Location + Width  bit1=0  base1=MSB of Input  bit0=freqBits  base0=LSB of Input  dbl_ovrd=off  block_type=slice
  Slice1 : xbsIndex_r4/Slice  nbits=freqBits  boolean_output=off  mode=Lower Bit Location + Width  bit1=0  base1=MSB of Input  bit0=0  base0=LSB of Input  dbl_ovrd=off  block_type=slice
  Terminator{,1..6,8} (8 alike) : Terminator
  block downconverter Scope : Scope  NumInputPorts=3
  block downconverter Scope1 : Scope  NumInputPorts=2
  block downconverter Scope2 : Scope  NumInputPorts=6
  block downconverter Scope3 : Scope  NumInputPorts=8
  DC_Out : Outport
  UC_out : Outport  Port=2
  wires:
  Relational/1 -> "DDS Compiler 6.0 "/1
  [freqBus] -> Register3/1
  Slice/1 -> Relational/2
  Slice1/1 -> Reinterpret2/1
  addrIn/1 -> [Addr], Relational1/1, Relational/1
  "DDS Compiler 6.0 "/2 -> Complex Multiplier 6.0 4/2, Delay/1
  "DDS Compiler 6.0 "/3 -> Complex Multiplier 6.0 4/3, Delay1/1
  Relational1/1 -> Register/2, Register1/2
  Register1/1 -> Gateway Out15/1, Complex Multiplier 6.0 4/6
  Register/1 -> Relational2/2, Gateway Out16/1, Complex Multiplier 6.0 4/5
  "DDS Compiler 6.0 "/1 -> Complex Multiplier 6.0 4/1, Complex Multiplier 6.0 4/4
  Delay/1 -> Mult1/1, Gateway Out8/1, [UC_LO_Q]
  Delay1/1 -> Gateway Out7/1, Mult8/1, [UC_LO_I]
  "CIC Compiler 4.0 "/3 -> Gateway Out31/1, Scale1/1
  CIC Compiler 4.0 3/3 -> Scale4/1
  CIC Compiler 4.0 2/3 -> Scale3/1
  CIC Compiler 4.0 1/3 -> Gateway Out30/1, Scale2/1
  Mux2/1 -> Demux1/1, DC_Out/1
  Scale4/1 -> Gateway Out13/1, Mux1/2  "mdREF_I"
  Scale3/1 -> Gateway Out14/1, Mux1/1  "mdREF_Q"
  Scale2/1 -> Mux/2  "mdADC_I"
  Scale1/1 -> Mux/1  "mdADC_Q"
  Constant/1 -> CIC Compiler 4.0 1/1, CIC Compiler 4.0 3/1, CIC Compiler 4.0 2/1, "CIC Compiler 4.0 "/1
  Mux1/1 -> Mux2/2
  Mux/1 -> Mux2/1
  "CIC Compiler 4.0 "/1 -> Terminator/1
  CIC Compiler 4.0 1/1 -> Terminator2/1
  CIC Compiler 4.0 1/2 -> Terminator3/1
  CIC Compiler 4.0 2/1 -> Terminator4/1
  CIC Compiler 4.0 2/2 -> Terminator5/1
  Complex Multiplier 6.0 4/1 -> Terminator8/1
  Bus Selector/2 -> Register/1  "<dPhiQ>"
  Bus Selector/3 -> Register1/1  "<dPhiI>"
  Reinterpret2/1 -> "DDS Compiler 6.0 "/2
  [dphiBus] -> Bus Selector/1
  Bus Selector/1 -> Relational1/2  "<channel>"
  Demux1/1 -> Gateway Out3/1
  Demux1/2 -> Gateway Out4/1
  Demux1/3 -> Gateway Out5/1
  Demux1/4 -> Gateway Out6/1
  Gateway Out6/1 -> Mux5/2
  Gateway Out5/1 -> Mux5/1
  Gateway Out4/1 -> Mux4/2
  Gateway Out3/1 -> Mux4/1
  Mux4/1 -> block downconverter Scope/1
  Mux5/1 -> block downconverter Scope/2
  Convert2/1 -> Gateway Out9/1, Mult9/2
  Convert1/1 -> Gateway Out10/1, Mult2/2
  Gateway Out10/1 -> Mux7/2
  Gateway Out9/1 -> Mux7/1
  Gateway Out8/1 -> Mux6/2
  Gateway Out7/1 -> Mux6/1
  Mux6/1 -> DLO1 scope/1
  Mux7/1 -> DLO1 scope/2
  Gateway Out16/1 -> Display4/1
  Gateway Out15/1 -> Display3/1
  Constant1/1 -> Mux13/2
  [Ampl0] -> Mux13/3
  Mux13/1 -> Gateway Out20/1, Mult9/1, Mult2/1, Mult1/2, Mult8/2
  Constant2/1 -> Relational2/1
  Relational2/1 -> Mux13/1
  Gateway Out20/1 -> Display5/1
  Relational3/1 -> Inverter/1, "CIC Compiler 4.0 "/3, CIC Compiler 4.0 1/3, CIC Compiler 4.0 3/3, CIC Compiler 4.0 2/3
  [Addr] -> Relational3/2
  synchIn/1 -> Relational3/1
  Gateway Out21/1 -> block downconverter Scope1/1
  Counter/1 -> Gateway Out22/1
  Gateway Out22/1 -> block downconverter Scope/3, block downconverter Scope1/2
  Inverter/1 -> Counter/1, Gateway Out21/1
  ADC_IQ_in/1 -> Demux2/1
  Demux2/1 -> Gateway Out29/1, Complex Multiplier 6.0 1/2
  Demux2/2 -> Gateway Out24/1, Complex Multiplier 6.0 1/3
  Complex Multiplier 6.0 1/2 -> "CIC Compiler 4.0 "/2, Gateway Out28/1
  Complex Multiplier 6.0 1/3 -> Gateway Out27/1, CIC Compiler 4.0 1/2
  [UC_LO_Q] -> Gateway Out26/1, Complex Multiplier 6.0 2/5, Complex Multiplier 6.0 1/5
  [UC_LO_I] -> Gateway Out25/1, Complex Multiplier 6.0 2/6, Complex Multiplier 6.0 1/6
  Complex Multiplier 6.0 2/3 -> CIC Compiler 4.0 3/2, Gateway Out12/1
  Complex Multiplier 6.0 2/2 -> CIC Compiler 4.0 2/2, Gateway Out11/1
  Demux3/1 -> Register8/1
  Demux3/2 -> Register9/1
  REF_IQ_in1/1 -> Demux3/1
  Constant3/1 -> Complex Multiplier 6.0 1/1, Complex Multiplier 6.0 1/4, Complex Multiplier 6.0 2/4, Complex Multiplier 6.0 2/1
  CIC Compiler 4.0 3/1 -> Terminator1/1
  CIC Compiler 4.0 3/2 -> Terminator6/1
  Mult1/1 -> Register7/1, Gateway Out19/1
  Mult8/1 -> Register6/1, Gateway Out18/1
  Mult2/1 -> Register5/1, Gateway Out17/1
  Mult9/1 -> Register4/1, Gateway Out23/1
  Mux3/1 -> DLO1 scope1/1
  Mux8/1 -> DLO1 scope1/2
  Complex Multiplier 6.0 4/3 -> Convert2/1
  Complex Multiplier 6.0 4/2 -> Convert1/1
  Gateway Out1/1 -> block downconverter Scope2/1
  Gateway Out2/1 -> block downconverter Scope2/2
  Gateway Out11/1 -> block downconverter Scope2/3
  Gateway Out12/1 -> block downconverter Scope2/4
  Gateway Out13/1 -> block downconverter Scope2/5
  Gateway Out14/1 -> block downconverter Scope2/6
  Gateway Out17/1 -> Mux8/2
  Gateway Out23/1 -> Mux8/1
  Gateway Out19/1 -> Mux3/2
  Gateway Out18/1 -> Mux3/1
  Gateway Out24/1 -> block downconverter Scope3/1
  Gateway Out29/1 -> block downconverter Scope3/2
  Gateway Out25/1 -> block downconverter Scope3/3
  Gateway Out26/1 -> block downconverter Scope3/4
  Gateway Out27/1 -> block downconverter Scope3/5
  Gateway Out28/1 -> block downconverter Scope3/6
  Gateway Out30/1 -> block downconverter Scope3/7
  Gateway Out31/1 -> block downconverter Scope3/8
  Register3/1 -> Slice1/1, Slice/1
  Register8/1 -> Gateway Out2/1, Complex Multiplier 6.0 2/2
  Register9/1 -> Gateway Out1/1, Complex Multiplier 6.0 2/3
  Bus Creator/1 -> UC_out/1
  Register4/1 -> Bus Creator/4  "UC_out_Ip"
  Register5/1 -> Bus Creator/3  "UC_out_Qp"
  Register6/1 -> Bus Creator/2  "UC_out_I"
  Register7/1 -> Bus Creator/1  "UC_out_Q"
